simulink model "MotorModelo6v"  (R2025a)
settings: Solver=VariableStepAuto  StartTime=0.0  StopTime=20  RelTol=1e-3
values from neighbouring files (symbols this model uses):
  B = p0(2)    [DC_Motor.m]    (also in Parametros_Motor.m = 0.0082235)
  J = p0(1)    [DC_Motor.m]    (also in Parametros_Motor.m = 0.0011997)
  Ka = p0(3)    [DC_Motor.m]    (also in Parametros_Motor.m = 0.63643)
  Km = p0(4)    [DC_Motor.m]    (also in Parametros_Motor.m = 0.63643)
  L = p0(6)    [DC_Motor.m]    (also in Parametros_Motor.m = 0.0043199)
  R = p0(5)    [DC_Motor.m]    (also in Parametros_Motor.m = 8.64)
libraries: cstblocks x1
settings Model: Creator=Sergio  LastModifiedBy=mario
settings SolverCC: AlgebraicLoopSolver=TrustRegion
settings DataIOCC: ReturnWorkspaceOutputs=off
settings DebuggingCC: UnconnectedInputMsg=warning  UnconnectedOutputMsg=warning  UnconnectedLineMsg=warning  ArithmeticOperatorsInVariantConditions=warning
settings ModelReferenceCC: EnableRefExpFcnMdlSchedulingChecks=on
settings SFSimCC: SimUseLocalCustomCode=off  CustomCodeUndefinedFunction=UseInterfaceOnly
settings RTWCC: RTWUseLocalCustomCode=off  GPUComputeCapability=3.5  DLArmComputeVersion=19.05

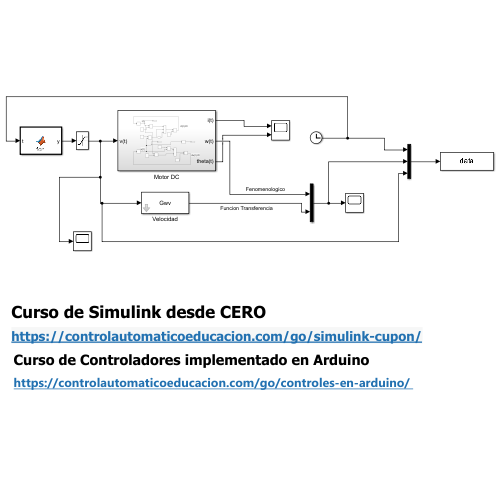
[thumbnail: Simulink's stored preview of the top-level diagram]
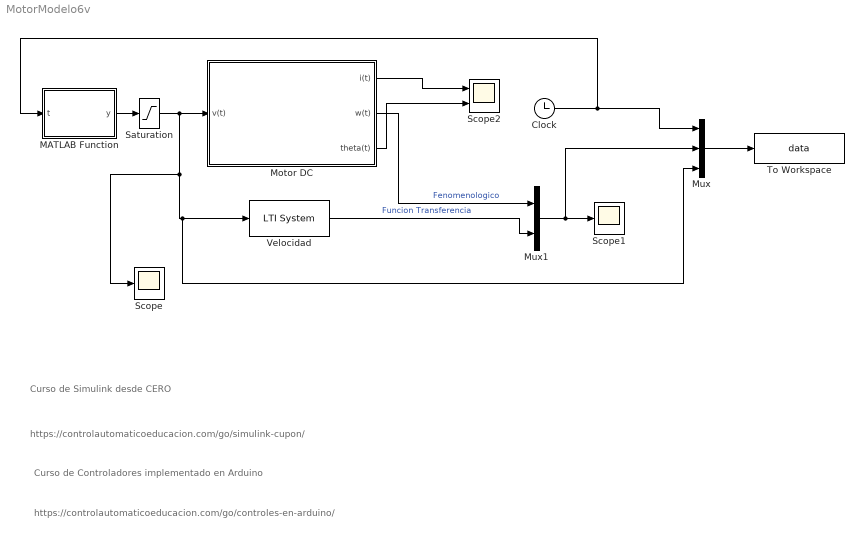
== system MotorModelo6v ==
  note: https://controlautomaticoeducacion.com/go/controles-en-arduino/
  note: Curso de Simulink desde CERO
  note: Curso de Controladores implementado en Arduino
  note: https://controlautomaticoeducacion.com/go/simulink-cupon/
  Clock : Clock
  MATLAB Function : MATLAB Function  TreatAsAtomicUnit=on
  Motor DC : Subsystem
  Mux : Mux  Inputs=3
  Mux1 : Mux  Inputs=2
  Saturation : Saturate  UpperLimit=12  LowerLimit=0
  Scope : Scope
      settings: ActiveDisplayYMinimum=-1  ActiveDisplayYMaximum=1
  Scope1 : Scope
      settings: ActiveDisplayYMinimum=-1.80104  ActiveDisplayYMaximum=16.20351
  Scope2 : Scope  NumInputPorts=2
      settings: ActiveDisplayYMinimum=-12.536708336283766  ActiveDisplayYMaximum=102.34825136023548  DataLoggingVariableName=ScopeData2
  To Workspace : ToWorkspace  VariableName=data  SampleTime=0.05
  Velocidad : cstblocks/LTI System  sys=Gwv  IC=[]  PadeOrder=0
  wires:
  Motor DC/2(w(t)) -> Mux1/1  "Fenomenologico"
  Velocidad/1 -> Mux1/2  "Funcion Transferencia"
  MATLAB Function/1(y) -> Saturation/1
  Saturation/1 -> Scope/1, Mux/3, Velocidad/1, Motor DC/1(v(t))
  Mux/1 -> To Workspace/1
  Clock/1 -> MATLAB Function/1(t), Mux/1
  Mux1/1 -> Mux/2, Scope1/1
  Motor DC/1(i(t)) -> Scope2/1
  Motor DC/3(theta(t)) -> Scope2/2

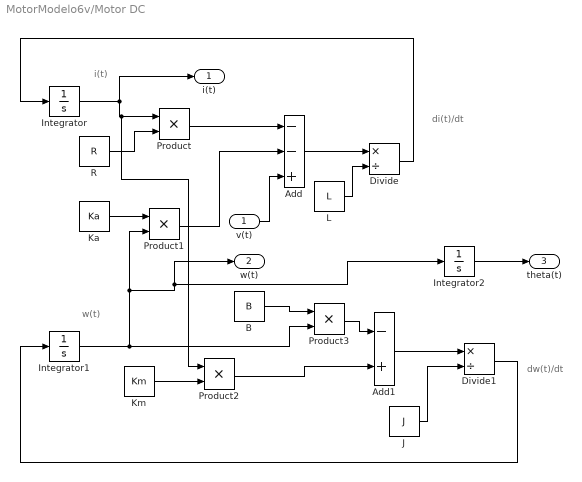
== system MotorModelo6v/Motor DC ==
  note: i(t)
  note: w(t)
  note: di(t)/dt
  note: dw(t)/dt
  v(t) : Inport
  Add : Sum  Inputs=--+
  Add1 : Sum  Inputs=-+
  B : Constant  Value=B
  Divide : Product  Inputs=*/
  Divide1 : Product  Inputs=*/
  Integrator : Integrator
  Integrator1 : Integrator
  Integrator2 : Integrator
  J : Constant  Value=J
  Ka : Constant  Value=Ka
  Km : Constant  Value=Km
  L : Constant  Value=L
  Product{,1..3} (4 alike) : Product
  R : Constant  Value=R
  i(t) : Outport  VectorParamsAs1DForOutWhenUnconnected=off
  w(t) : Outport  Port=2  VectorParamsAs1DForOutWhenUnconnected=off
  theta(t) : Outport  Port=3  VectorParamsAs1DForOutWhenUnconnected=off
  wires:
  Divide/1 -> Integrator/1
  Integrator/1 -> i(t)/1, Product2/1, Product/1
  Integrator1/1 -> Product3/2, w(t)/1, Integrator2/1, Product1/2
  R/1 -> Product/2
  Add1/1 -> Divide1/1
  v(t)/1 -> Add/3
  Ka/1 -> Product1/1
  J/1 -> Divide1/2
  Product3/1 -> Add1/1
  Product1/1 -> Add/2
  Add/1 -> Divide/1
  Product/1 -> Add/1
  L/1 -> Divide/2
  Divide1/1 -> Integrator1/1
  Integrator2/1 -> theta(t)/1
  B/1 -> Product3/1
  Km/1 -> Product2/2
  Product2/1 -> Add1/2

== matlab function MotorModelo6v/MATLAB Function ==
  data: t input; y output
function y = fcn(t)
    if t < 2
        y = 0;
    elseif t < 4
        y = 11.44;
    elseif t < 6
        y = 0;
    elseif t < 8
        y = 9.00;
    elseif t < 10
        y = 0;
    elseif t < 12
        y = 6.74;
    elseif t < 14
        y = 0;
    elseif t < 16
        y = 4.52;
    elseif t < 18
        y = 0;
    else
        y = 2.31;
    end
